simulink model "Air_Drag"  (R2023b)
settings: Solver=VariableStepAuto  StartTime=0.0  StopTime=T_1orbit  RelTol=1e-6
values from neighbouring files (symbols this model uses):
  a = 6939    [Air_Drag_script.m]    (also in main.m = 6939.063; main_group24.m = 6978)
  A0 = eye(3)    [Air_Drag_script.m]
  A1 = 6e-2    (= 0.06)    [Air_Drag_script.m]
  A10 = 12e-2    (= 0.12)    [Air_Drag_script.m]
  A2 = 6e-2    (= 0.06)    [Air_Drag_script.m]
  A3 = 4e-2    (= 0.04)    [Air_Drag_script.m]
  A4 = 6e-2    (= 0.06)    [Air_Drag_script.m]
  A5 = 6e-2    (= 0.06)    [Air_Drag_script.m]
  A6 = 4e-2    (= 0.04)    [Air_Drag_script.m]
  A7 = 12e-2    (= 0.12)    [Air_Drag_script.m]
  A8 = 12e-2    (= 0.12)    [Air_Drag_script.m]
  A9 = 12e-2    (= 0.12)    [Air_Drag_script.m]
  cd = 2.2    [Air_Drag_script.m]
  e = 0    [Air_Drag_script.m]    (also in main.m = 0.001304; main_group24.m)
  i = deg2rad(97.5307)    [Air_Drag_script.m]    (also in main.m; main_group24.m = deg2rad(98))
  Ix = J(1,1)    [Air_Drag_script.m]    (also in data_mass.m = 0.0755003333333; main.m = 0.057749855; main_group24.m = 0.0755003333333)
  Iy = J(2,2)    [Air_Drag_script.m]    (also in data_mass.m = 0.0755003333333; main.m = 0.04143542; main_group24.m = 0.0755003333333)
  Iz = J(3,3)    [Air_Drag_script.m]    (also in data_mass.m = 0.055; main.m = 0.024624309; main_group24.m = 0.055)
  n = 0.0011    [Air_Drag_script.m]    (also in main.m = sqrt(mu/a^3); main_group24.m = sqrt(mu/a^3))
  n1 = [1 0 0]'    [Air_Drag_script.m]
  n10 = -n9    [Air_Drag_script.m]
  n2 = [0 1 0]'    [Air_Drag_script.m]
  n3 = [0 0 1]'    [Air_Drag_script.m]
  n4 = -n1    [Air_Drag_script.m]
  n5 = -n2    [Air_Drag_script.m]
  n6 = -n3    [Air_Drag_script.m]
  n7 = [1 0 0]'    [Air_Drag_script.m]
  n8 = -n7    [Air_Drag_script.m]
  n9 = [1 0 0]'    [Air_Drag_script.m]
  q0 = [ 1 1 1 1 ]'    [Air_Drag_script.m]    (also in main_group24.m = [0 0 0 1]')
  r1 = [10 0 0]'*1e-2    [Air_Drag_script.m]
  r10 = r9    [Air_Drag_script.m]
  r2 = [0,10,0]'*1e-2    [Air_Drag_script.m]
  r3 = [0,0,10]'*1e-2    [Air_Drag_script.m]
  r4 = -r1    [Air_Drag_script.m]
  r5 = -r2    [Air_Drag_script.m]
  r6 = -r3    [Air_Drag_script.m]
  r7 = [0,0,45]'*1e-2    [Air_Drag_script.m]
  r8 = r7    [Air_Drag_script.m]
  r9 = [0,0,-45]'*1e-2    [Air_Drag_script.m]
  rho_air = 1.65e-13    [Air_Drag_script.m]    (also in main_group24.m = 6.967e-13)
  w0 = [0 0 0]'    [Air_Drag_script.m]    (also in main.m = [wx0; wy0; wz0]; main_group24.m = [wx0; wy0; wz0])
  w_earth = [0 0 7.2921e-5]'    [Air_Drag_script.m]
libraries: matrix_library x12, vrlib x10
settings Model: Creator=hp  LastModifiedBy=hp

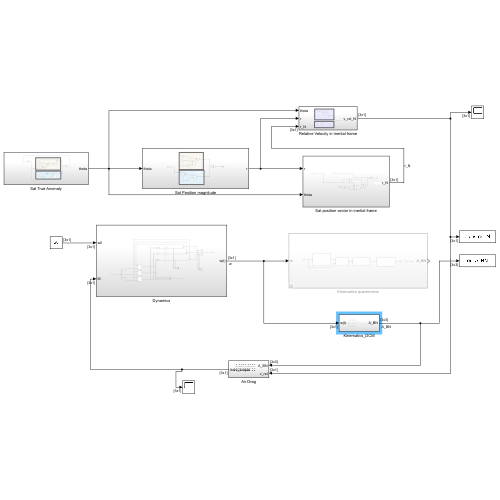
[thumbnail: Simulink's stored preview of the top-level diagram]
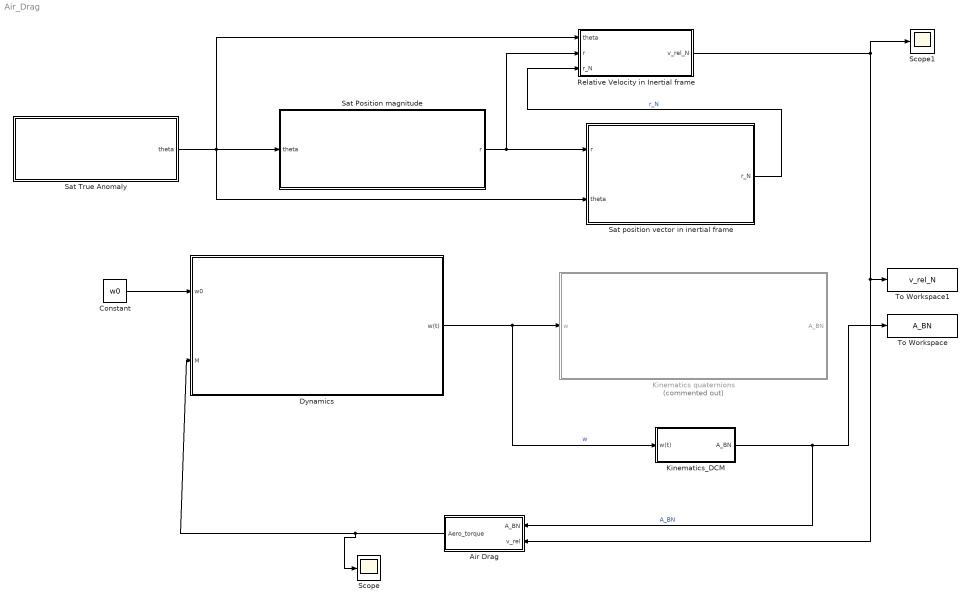
== system Air_Drag ==
  Air Drag : Subsystem
  Constant : Constant  Value=w0  VectorParams1D=off
  Dynamics : Subsystem
  Kinematics quaternions : Subsystem  Commented=on
  Kinematics_DCM : Subsystem
  Relative Velocity in Inertial frame : Subsystem
  Sat Position magnitude : Subsystem
  Sat True Anomaly : Subsystem
  Sat position vector in inertial frame : Subsystem
  Scope : Scope
  Scope1 : Scope
  To Workspace : ToWorkspace  VariableName=A_BN  SaveFormat=Timeseries  SampleTime=-1
  To Workspace1 : ToWorkspace  VariableName=v_rel_N  SaveFormat=Timeseries  SampleTime=-1
  wires:
  Sat True Anomaly/1(theta) -> Relative Velocity in Inertial frame/1(theta), Sat position vector in inertial frame/2(theta), Sat Position magnitude/1(theta)
  Sat Position magnitude/1(r) -> Sat position vector in inertial frame/1(r), Relative Velocity in Inertial frame/2(r)
  Sat position vector in inertial frame/1(r_N) -> Relative Velocity in Inertial frame/3(r_N)  "r_N"
  Dynamics/1(w(t)) -> Kinematics_DCM/1(w(t)), Kinematics quaternions/1(w)  "w"
  Constant/1 -> Dynamics/1(w0)
  Relative Velocity in Inertial frame/1(v_rel_N) -> To Workspace1/1, Air Drag/2(v_rel), Scope1/1
  Air Drag/1(Aero_torque) -> Scope/1, Dynamics/2(M)
  Kinematics_DCM/1(A_BN) -> Air Drag/1(A_BN), To Workspace/1  "A_BN"

== system Air_Drag/Air Drag ==
  A_BN : Inport
  v_rel : Inport  Port=2
  Sum of Elements : Sum  Inputs=++++++++++
  T1 : Subsystem
  T10 : Subsystem
  T2 : Subsystem
  T3 : Subsystem
  T4 : Subsystem
  T5 : Subsystem
  T6 : Subsystem
  T7 : Subsystem
  T8 : Subsystem
  T9 : Subsystem
  Aero_torque : Outport
  wires:
  Sum of Elements/1 -> Aero_torque/1
  v_rel/1 -> T10/1(v_rel_N), T7/1(v_rel_N), T6/1(v_rel_N), T2/1(v_rel_N), T1/1(v_rel_N), T3/1(v_rel_N), T4/1(v_rel_N), T5/1(v_rel_N), T8/1(v_rel_N), T9/1(v_rel_N)  "v_rel_N"
  A_BN/1 -> T8/2(A_BN), T5/2(A_BN), T4/2(A_BN), T2/2(A_BN), T1/2(A_BN), T3/2(A_BN), T6/2(A_BN), T7/2(A_BN), T9/2(A_BN), T10/2(A_BN)
  T1/1(Out1) -> Sum of Elements/1
  T2/1(Out1) -> Sum of Elements/2
  T3/1(Out1) -> Sum of Elements/3
  T4/1(Out1) -> Sum of Elements/4
  T5/1(Out1) -> Sum of Elements/5
  T6/1(Out1) -> Sum of Elements/6
  T7/1(Out1) -> Sum of Elements/7
  T8/1(Out1) -> Sum of Elements/8
  T9/1(Out1) -> Sum of Elements/9
  T10/1(Out1) -> Sum of Elements/10

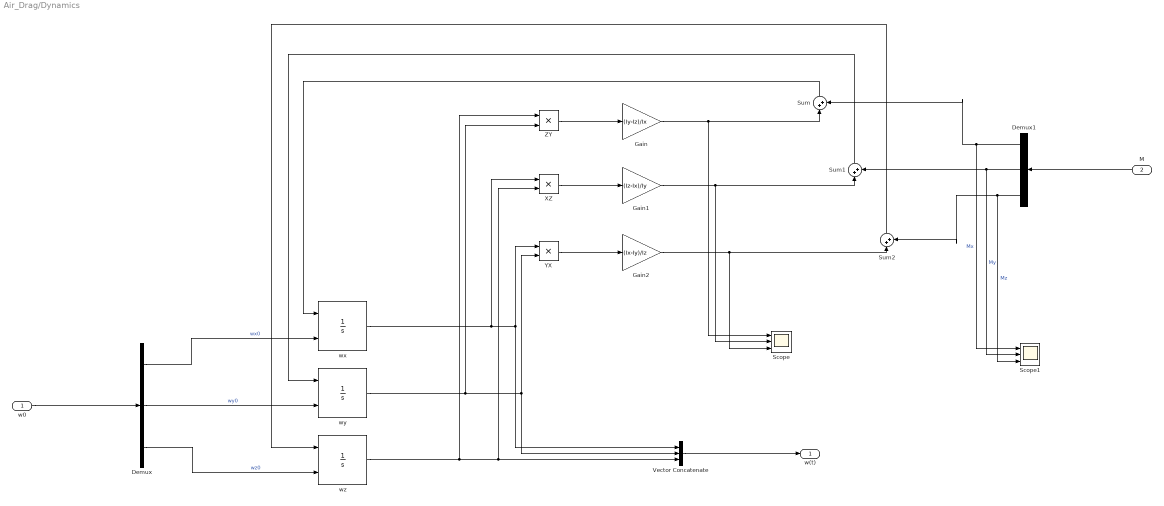
== system Air_Drag/Dynamics ==
  w0 : Inport
  M : Inport  Port=2
  Demux : Demux  Outputs=3
  Demux1 : Demux  Outputs=3
  Gain : Gain  Gain=(Iy-Iz)/Ix
  Gain1 : Gain  Gain=(Iz-Ix)/Iy
  Gain2 : Gain  Gain=(Ix-Iy)/Iz
  Scope : Scope  NumInputPorts=3
  Scope1 : Scope  NumInputPorts=3
  Sum : Sum  Inputs=|++
  Sum1 : Sum  Inputs=|++
  Sum2 : Sum  Inputs=|++
  Vector Concatenate : Concatenate  NumInputs=3  Mode=Multidimensional array
  XZ : Product
  YX : Product
  ZY : Product
  wx : Integrator  InitialConditionSource=external
  wy : Integrator  InitialConditionSource=external
  wz : Integrator  InitialConditionSource=external
  w(t) : Outport
  wires:
  XZ/1 -> Gain1/1
  Demux/2 -> wy/2  "wy0"
  wx/1 -> XZ/1, Vector Concatenate/1, YX/1
  w0/1 -> Demux/1
  wy/1 -> Vector Concatenate/2, YX/2, ZY/2
  Demux/1 -> wx/2  "wx0"
  wz/1 -> ZY/1, Vector Concatenate/3, XZ/2
  YX/1 -> Gain2/1
  Demux/3 -> wz/2  "wz0"
  ZY/1 -> Gain/1
  Vector Concatenate/1 -> w(t)/1
  Gain2/1 -> Scope/3, Sum2/1
  Gain1/1 -> Scope/2, Sum1/1
  Gain/1 -> Scope/1, Sum/1
  Sum/1 -> wx/1
  Sum1/1 -> wy/1
  Sum2/1 -> wz/1
  Demux1/1 -> Scope1/1, Sum/2  "Mx"
  Demux1/2 -> Scope1/2, Sum1/2  "My"
  Demux1/3 -> Sum2/2, Scope1/3  "Mz"
  M/1 -> Demux1/1

== system Air_Drag/Kinematics quaternions ==
  w : Inport
  A_BN from q_vect : MATLAB Function  TreatAsAtomicUnit=on
  Create Omega Matrix : Subsystem
  Kinematics_quaternions : Subsystem
  Normalizer : Subsystem
  w_at_matrix : Subsystem
  A_BN : Outport
  wires:
  Kinematics_quaternions/1(q_vect) -> A_BN from q_vect/1(q_vect)
  A_BN from q_vect/1(A_BN) -> Normalizer/1(A_BN)
  w/1 -> Create Omega Matrix/2(w), w_at_matrix/1(w(t))
  Create Omega Matrix/1(Omega) -> Kinematics_quaternions/1(Omega)  "Omega"
  w_at_matrix/1("[-w^]") -> Create Omega Matrix/1("[w^]")  "[-w^]"
  Normalizer/1(Out1) -> A_BN/1

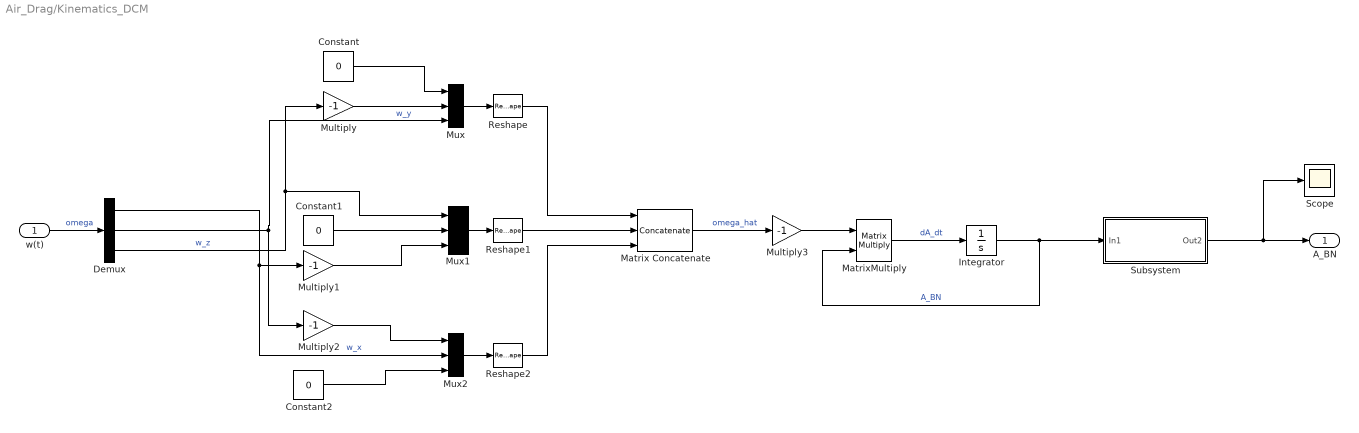
== system Air_Drag/Kinematics_DCM ==
  w(t) : Inport
  Constant : Constant  Value=0
  Constant1 : Constant  Value=0
  Constant2 : Constant  Value=0
  Demux : Demux  Outputs=3
  Integrator : Integrator  InitialCondition=A0
  Matrix Concatenate : Concatenate  NumInputs=3  Mode=Multidimensional array
  MatrixMultiply : Product  Multiplication=Matrix(*)
  Multiply{,1..3} (4 alike) : Gain  Gain=-1
  Mux : Mux  Inputs=3
  Mux1 : Mux  Inputs=3
  Mux2 : Mux  Inputs=3
  Reshape : Reshape  OutputDimensionality=Row vector (2-D)
  Reshape1 : Reshape  OutputDimensionality=Row vector (2-D)
  Reshape2 : Reshape  OutputDimensionality=Row vector (2-D)
  Scope : Scope
  Subsystem : Subsystem
  A_BN : Outport
  wires:
  w(t)/1 -> Demux/1  "omega"
  MatrixMultiply/1 -> Integrator/1  "dA_dt"
  Matrix Concatenate/1 -> Multiply3/1  "omega_hat"
  Constant/1 -> Mux/1
  Demux/3 -> Mux1/1, Multiply/1  "w_z"
  Multiply/1 -> Mux/2
  Demux/2 -> Mux/3, Multiply2/1  "w_y"
  Constant1/1 -> Mux1/2
  Demux/1 -> Mux2/2, Multiply1/1  "w_x"
  Multiply1/1 -> Mux1/3
  Constant2/1 -> Mux2/3
  Multiply2/1 -> Mux2/1
  Mux/1 -> Reshape/1
  Mux1/1 -> Reshape1/1
  Mux2/1 -> Reshape2/1
  Multiply3/1 -> MatrixMultiply/1
  Reshape/1 -> Matrix Concatenate/1
  Reshape1/1 -> Matrix Concatenate/2
  Reshape2/1 -> Matrix Concatenate/3
  Integrator/1 -> Subsystem/1(In1), MatrixMultiply/2  "A_BN"
  Subsystem/1(Out2) -> Scope/1, A_BN/1

== system Air_Drag/Relative Velocity in Inertial frame ==
  note: V_orbit
  note: V_atmosphere
  theta : Inport
  r : Inport  Port=2
  r_N : Inport  Port=3
  Constant : Constant  Value=n
  Constant3 : Constant  Value=w_earth  VectorParams1D=off
  Cos : Trigonometry  Operator=cos
  Cross Product : matrix_library/Cross Product
  Gain : Gain  Gain=-1
  Gain1 : Gain  Gain=cos(i)
  Gain2 : Gain  Gain=sin(i)
  Product : Product  Inputs=3
  Sin : Trigonometry
  Sum1 : Sum  Inputs=+-
  Vector Concatenate : Concatenate  NumInputs=3
  v_rel_N : Outport
  wires:
  Sum1/1 -> v_rel_N/1
  r_N/1 -> Cross Product/2
  Constant3/1 -> Cross Product/1
  Product/1 -> Sum1/1
  Cross Product/1 -> Sum1/2
  r/1 -> Product/2
  Constant/1 -> Product/3
  theta/1 -> Cos/1, Sin/1
  Gain/1 -> Vector Concatenate/1
  Gain1/1 -> Vector Concatenate/2
  Gain2/1 -> Vector Concatenate/3
  Cos/1 -> Gain2/1, Gain1/1
  Sin/1 -> Gain/1
  Vector Concatenate/1 -> Product/1

== system Air_Drag/Sat Position magnitude ==
  note: 1+e cos(theta)
  note: a(1-e^2)
  note: Denominator
  note: Numerator
  theta : Inport
  Constant : Constant  Value=a
  Constant1 : Constant
  Constant3 : Constant  Value=e
  Constant4 : Constant
  Constant5 : Constant  Value=e
  Cos : Trigonometry  Operator=cos
  Divide : Product  Inputs=*/
  Product : Product
  Product1 : Product
  Square1 : Math  Operator=square
  Sum : Sum
  Sum1 : Sum  Inputs=+-
  r : Outport
  wires:
  Product1/1 -> Sum/1
  Sum1/1 -> Product/2
  Constant1/1 -> Sum1/1
  Sum/1 -> Divide/2
  Square1/1 -> Sum1/2
  Constant3/1 -> Product1/2
  Constant4/1 -> Sum/2
  Constant/1 -> Product/1
  Constant5/1 -> Square1/1
  Cos/1 -> Product1/1
  Product/1 -> Divide/1
  theta/1 -> Cos/1
  Divide/1 -> r/1

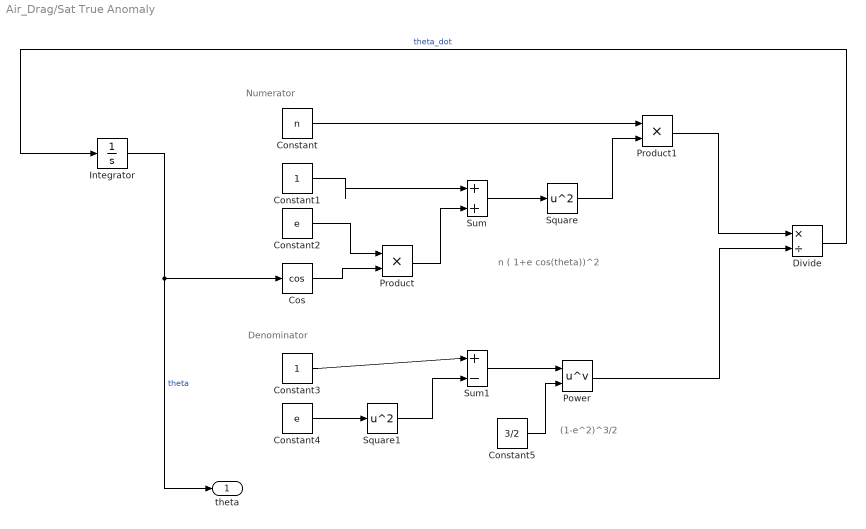
== system Air_Drag/Sat True Anomaly ==
  note: (1-e^2)^3/2
  note: n ( 1+e cos(theta))^2
  note: Denominator
  note: Numerator
  Constant : Constant  Value=n
  Constant1 : Constant
  Constant2 : Constant  Value=e
  Constant3 : Constant
  Constant4 : Constant  Value=e
  Constant5 : Constant  Value=3/2
  Cos : Trigonometry  Operator=cos
  Divide : Product  Inputs=*/
  Integrator : Integrator
  Power : Math  Operator=pow
  Product : Product
  Product1 : Product
  Square : Math  Operator=square
  Square1 : Math  Operator=square
  Sum : Sum  Inputs=|++
  Sum1 : Sum  Inputs=|+-
  theta : Outport
  wires:
  Sum/1 -> Square/1
  Integrator/1 -> theta/1, Cos/1  "theta"
  Square/1 -> Product1/2
  Constant5/1 -> Power/2
  Constant3/1 -> Sum1/1
  Product1/1 -> Divide/1
  Constant/1 -> Product1/1
  Divide/1 -> Integrator/1  "theta_dot"
  Square1/1 -> Sum1/2
  Product/1 -> Sum/2
  Power/1 -> Divide/2
  Constant1/1 -> Sum/1
  Constant2/1 -> Product/1
  Constant4/1 -> Square1/1
  Cos/1 -> Product/2
  Sum1/1 -> Power/1

== system Air_Drag/Sat position vector in inertial frame ==
  note: r_N = r [cos(theta)
      | 		sin(theta)cos(i)
      | 		sin(theta)sin(i)]
  r : Inport
  theta : Inport  Port=2
  Cos : Trigonometry  Operator=cos
  Cos1 : Trigonometry  Operator=cos
  Orbit Inclination : Constant  Value=i
  Product : Product
  Product1 : Product
  Product2 : Product
  Sin : Trigonometry
  Sin1 : Trigonometry
  Vector Concatenate : Concatenate  NumInputs=3  Mode=Multidimensional array
  r_N : Outport
  wires:
  Sin/1 -> Product1/1, Product/1
  Product/1 -> Vector Concatenate/2
  Sin1/1 -> Product1/2
  r/1 -> Product2/1
  Orbit Inclination/1 -> Sin1/1, Cos1/1
  Vector Concatenate/1 -> Product2/2
  theta/1 -> Cos/1, Sin/1
  Cos/1 -> Vector Concatenate/1
  Cos1/1 -> Product/2
  Product1/1 -> Vector Concatenate/3
  Product2/1 -> r_N/1

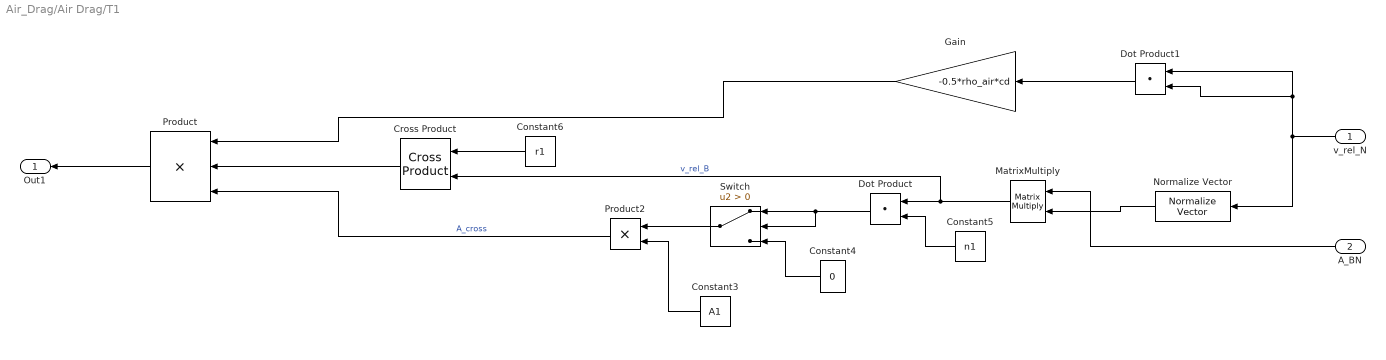
== system Air_Drag/Air Drag/T1 ==
  v_rel_N : Inport
  A_BN : Inport  Port=2
  Constant3 : Constant  Value=A1
  Constant4 : Constant  Value=0
  Constant5 : Constant  Value=n1  VectorParams1D=off
  Constant6 : Constant  Value=r1  VectorParams1D=off
  Cross Product : matrix_library/Cross Product
  Dot Product : DotProduct  OutDataTypeStr=Inherit: Inherit via internal rule
  Dot Product1 : DotProduct  OutDataTypeStr=Inherit: Inherit via internal rule
  Gain : Gain  Gain=-0.5*rho_air*cd
  MatrixMultiply : Product  Multiplication=Matrix(*)
  Normalize Vector : vrlib/Utilities/Normalize Vector  maxzero=0
  Product : Product  Inputs=3
  Product2 : Product
  Switch : Switch  Criteria=u2 > Threshold  SaturateOnIntegerOverflow=off  InputSameDT=off
  Out1 : Outport
  wires:
  MatrixMultiply/1 -> Cross Product/2, Dot Product/1  "v_rel_B"
  Constant4/1 -> Switch/3
  Dot Product/1 -> Switch/1, Switch/2
  v_rel_N/1 -> Dot Product1/2, Dot Product1/1, Normalize Vector/1
  Switch/1 -> Product2/1
  Constant6/1 -> Cross Product/1
  Constant5/1 -> Dot Product/2
  Constant3/1 -> Product2/2
  Gain/1 -> Product/1
  Dot Product1/1 -> Gain/1
  Cross Product/1 -> Product/2
  Product2/1 -> Product/3  "A_cross"
  Normalize Vector/1 -> MatrixMultiply/2
  A_BN/1 -> MatrixMultiply/1
  Product/1 -> Out1/1

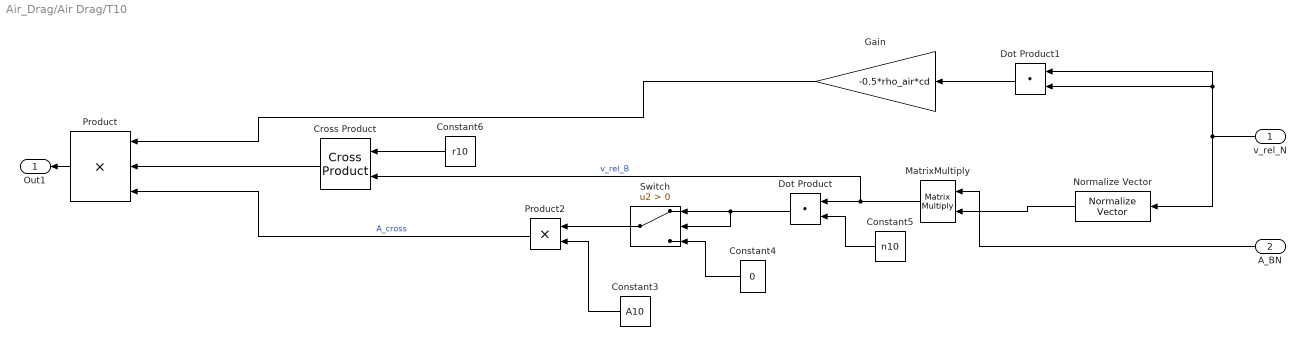
== system Air_Drag/Air Drag/T10 ==
  v_rel_N : Inport
  A_BN : Inport  Port=2
  Constant3 : Constant  Value=A10
  Constant4 : Constant  Value=0
  Constant5 : Constant  Value=n10  VectorParams1D=off
  Constant6 : Constant  Value=r10  VectorParams1D=off
  Cross Product : matrix_library/Cross Product
  Dot Product : DotProduct  OutDataTypeStr=Inherit: Inherit via internal rule
  Dot Product1 : DotProduct  OutDataTypeStr=Inherit: Inherit via internal rule
  Gain : Gain  Gain=-0.5*rho_air*cd
  MatrixMultiply : Product  Multiplication=Matrix(*)
  Normalize Vector : vrlib/Utilities/Normalize Vector  maxzero=0
  Product : Product  Inputs=3
  Product2 : Product
  Switch : Switch  Criteria=u2 > Threshold  SaturateOnIntegerOverflow=off  InputSameDT=off
  Out1 : Outport
  wires:
  Product/1 -> Out1/1
  A_BN/1 -> MatrixMultiply/1
  Normalize Vector/1 -> MatrixMultiply/2
  Product2/1 -> Product/3  "A_cross"
  Cross Product/1 -> Product/2
  Dot Product1/1 -> Gain/1
  Gain/1 -> Product/1
  Constant3/1 -> Product2/2
  Constant5/1 -> Dot Product/2
  Constant6/1 -> Cross Product/1
  Switch/1 -> Product2/1
  v_rel_N/1 -> Dot Product1/2, Dot Product1/1, Normalize Vector/1
  Dot Product/1 -> Switch/2, Switch/1
  Constant4/1 -> Switch/3
  MatrixMultiply/1 -> Dot Product/1, Cross Product/2  "v_rel_B"

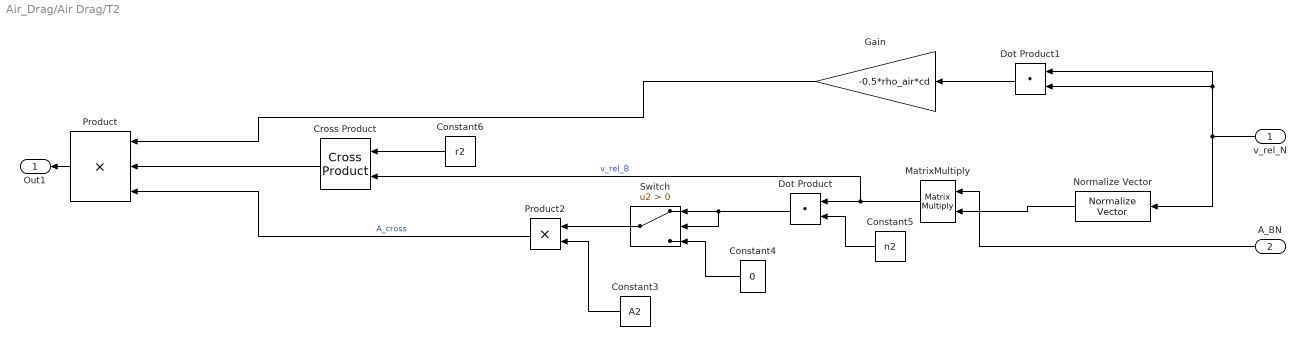
== system Air_Drag/Air Drag/T2 ==
  v_rel_N : Inport
  A_BN : Inport  Port=2
  Constant3 : Constant  Value=A2
  Constant4 : Constant  Value=0
  Constant5 : Constant  Value=n2  VectorParams1D=off
  Constant6 : Constant  Value=r2  VectorParams1D=off
  Cross Product : matrix_library/Cross Product
  Dot Product : DotProduct  OutDataTypeStr=Inherit: Inherit via internal rule
  Dot Product1 : DotProduct  OutDataTypeStr=Inherit: Inherit via internal rule
  Gain : Gain  Gain=-0.5*rho_air*cd
  MatrixMultiply : Product  Multiplication=Matrix(*)
  Normalize Vector : vrlib/Utilities/Normalize Vector  maxzero=0
  Product : Product  Inputs=3
  Product2 : Product
  Switch : Switch  Criteria=u2 > Threshold  SaturateOnIntegerOverflow=off  InputSameDT=off
  Out1 : Outport
  wires:
  Product/1 -> Out1/1
  A_BN/1 -> MatrixMultiply/1
  Normalize Vector/1 -> MatrixMultiply/2
  Product2/1 -> Product/3  "A_cross"
  Cross Product/1 -> Product/2
  Dot Product1/1 -> Gain/1
  Gain/1 -> Product/1
  Constant3/1 -> Product2/2
  Constant5/1 -> Dot Product/2
  Constant6/1 -> Cross Product/1
  Switch/1 -> Product2/1
  v_rel_N/1 -> Dot Product1/2, Dot Product1/1, Normalize Vector/1
  Dot Product/1 -> Switch/2, Switch/1
  Constant4/1 -> Switch/3
  MatrixMultiply/1 -> Dot Product/1, Cross Product/2  "v_rel_B"

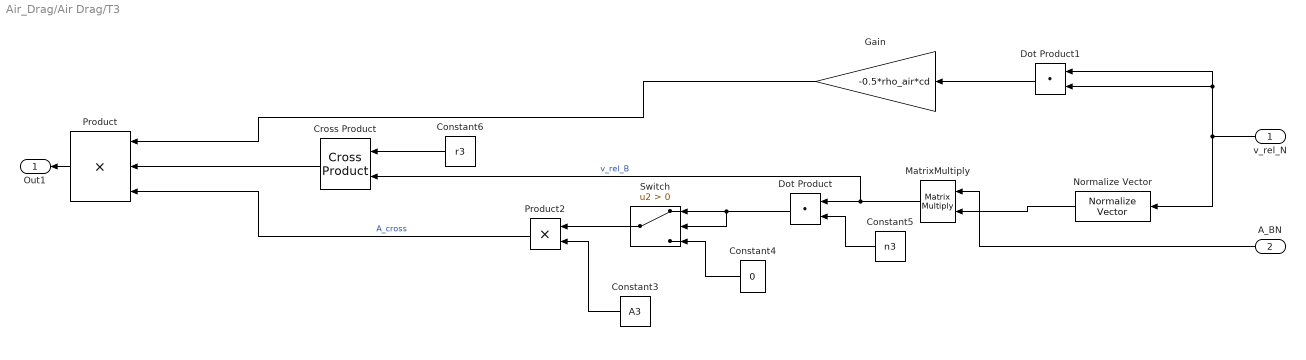
== system Air_Drag/Air Drag/T3 ==
  v_rel_N : Inport
  A_BN : Inport  Port=2
  Constant3 : Constant  Value=A3
  Constant4 : Constant  Value=0
  Constant5 : Constant  Value=n3  VectorParams1D=off
  Constant6 : Constant  Value=r3  VectorParams1D=off
  Cross Product : matrix_library/Cross Product
  Dot Product : DotProduct  OutDataTypeStr=Inherit: Inherit via internal rule
  Dot Product1 : DotProduct  OutDataTypeStr=Inherit: Inherit via internal rule
  Gain : Gain  Gain=-0.5*rho_air*cd
  MatrixMultiply : Product  Multiplication=Matrix(*)
  Normalize Vector : vrlib/Utilities/Normalize Vector  maxzero=0
  Product : Product  Inputs=3
  Product2 : Product
  Switch : Switch  Criteria=u2 > Threshold  SaturateOnIntegerOverflow=off  InputSameDT=off
  Out1 : Outport
  wires:
  MatrixMultiply/1 -> Cross Product/2, Dot Product/1  "v_rel_B"
  Constant4/1 -> Switch/3
  Dot Product/1 -> Switch/2, Switch/1
  v_rel_N/1 -> Dot Product1/2, Dot Product1/1, Normalize Vector/1
  Switch/1 -> Product2/1
  Constant6/1 -> Cross Product/1
  Constant5/1 -> Dot Product/2
  Constant3/1 -> Product2/2
  Gain/1 -> Product/1
  Dot Product1/1 -> Gain/1
  Cross Product/1 -> Product/2
  Product2/1 -> Product/3  "A_cross"
  Normalize Vector/1 -> MatrixMultiply/2
  A_BN/1 -> MatrixMultiply/1
  Product/1 -> Out1/1

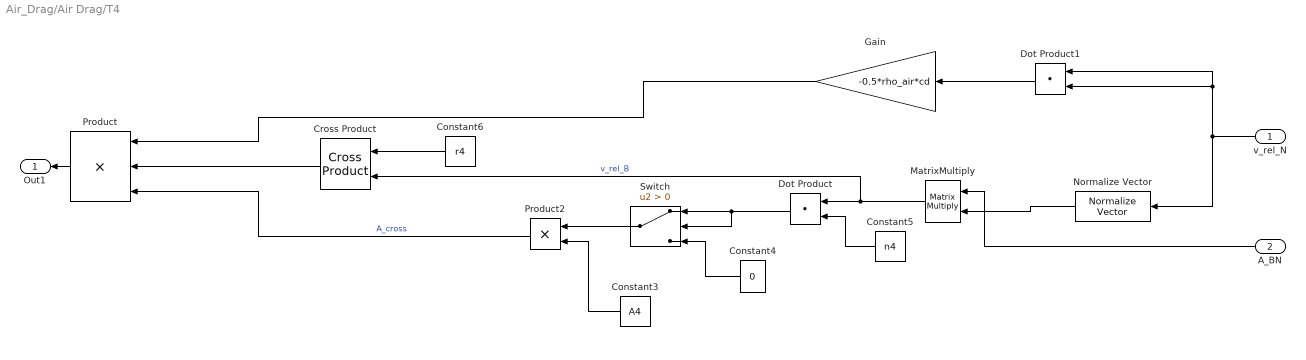
== system Air_Drag/Air Drag/T4 ==
  v_rel_N : Inport
  A_BN : Inport  Port=2
  Constant3 : Constant  Value=A4
  Constant4 : Constant  Value=0
  Constant5 : Constant  Value=n4  VectorParams1D=off
  Constant6 : Constant  Value=r4  VectorParams1D=off
  Cross Product : matrix_library/Cross Product
  Dot Product : DotProduct  OutDataTypeStr=Inherit: Inherit via internal rule
  Dot Product1 : DotProduct  OutDataTypeStr=Inherit: Inherit via internal rule
  Gain : Gain  Gain=-0.5*rho_air*cd
  MatrixMultiply : Product  Multiplication=Matrix(*)
  Normalize Vector : vrlib/Utilities/Normalize Vector  maxzero=0
  Product : Product  Inputs=3
  Product2 : Product
  Switch : Switch  Criteria=u2 > Threshold  SaturateOnIntegerOverflow=off  InputSameDT=off
  Out1 : Outport
  wires:
  Product/1 -> Out1/1
  A_BN/1 -> MatrixMultiply/1
  Normalize Vector/1 -> MatrixMultiply/2
  Product2/1 -> Product/3  "A_cross"
  Cross Product/1 -> Product/2
  Dot Product1/1 -> Gain/1
  Gain/1 -> Product/1
  Constant3/1 -> Product2/2
  Constant5/1 -> Dot Product/2
  Constant6/1 -> Cross Product/1
  Switch/1 -> Product2/1
  Dot Product/1 -> Switch/2, Switch/1
  Constant4/1 -> Switch/3
  MatrixMultiply/1 -> Dot Product/1, Cross Product/2  "v_rel_B"
  v_rel_N/1 -> Dot Product1/2, Dot Product1/1, Normalize Vector/1

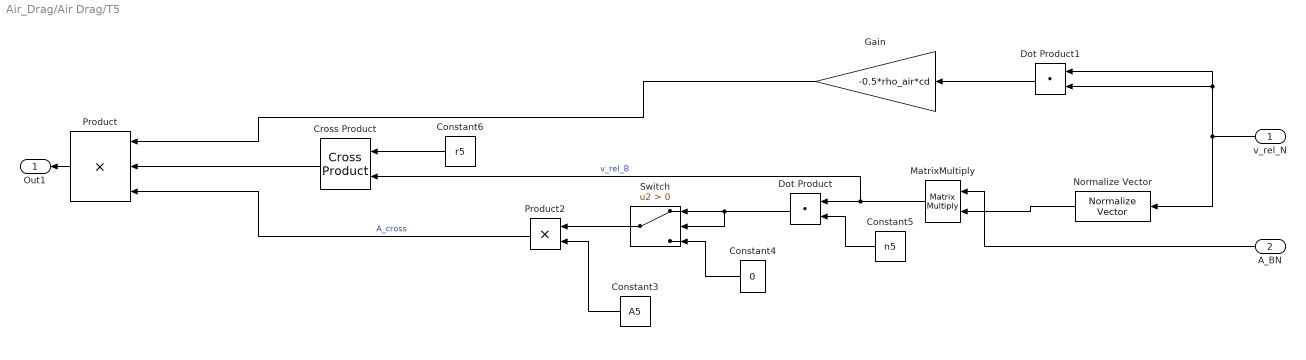
== system Air_Drag/Air Drag/T5 ==
  v_rel_N : Inport
  A_BN : Inport  Port=2
  Constant3 : Constant  Value=A5
  Constant4 : Constant  Value=0
  Constant5 : Constant  Value=n5  VectorParams1D=off
  Constant6 : Constant  Value=r5  VectorParams1D=off
  Cross Product : matrix_library/Cross Product
  Dot Product : DotProduct  OutDataTypeStr=Inherit: Inherit via internal rule
  Dot Product1 : DotProduct  OutDataTypeStr=Inherit: Inherit via internal rule
  Gain : Gain  Gain=-0.5*rho_air*cd
  MatrixMultiply : Product  Multiplication=Matrix(*)
  Normalize Vector : vrlib/Utilities/Normalize Vector  maxzero=0
  Product : Product  Inputs=3
  Product2 : Product
  Switch : Switch  Criteria=u2 > Threshold  SaturateOnIntegerOverflow=off  InputSameDT=off
  Out1 : Outport
  wires:
  MatrixMultiply/1 -> Cross Product/2, Dot Product/1  "v_rel_B"
  Constant4/1 -> Switch/3
  Dot Product/1 -> Switch/2, Switch/1
  Switch/1 -> Product2/1
  Constant6/1 -> Cross Product/1
  Constant5/1 -> Dot Product/2
  Constant3/1 -> Product2/2
  Gain/1 -> Product/1
  Dot Product1/1 -> Gain/1
  Cross Product/1 -> Product/2
  Product2/1 -> Product/3  "A_cross"
  Normalize Vector/1 -> MatrixMultiply/2
  A_BN/1 -> MatrixMultiply/1
  Product/1 -> Out1/1
  v_rel_N/1 -> Dot Product1/2, Dot Product1/1, Normalize Vector/1

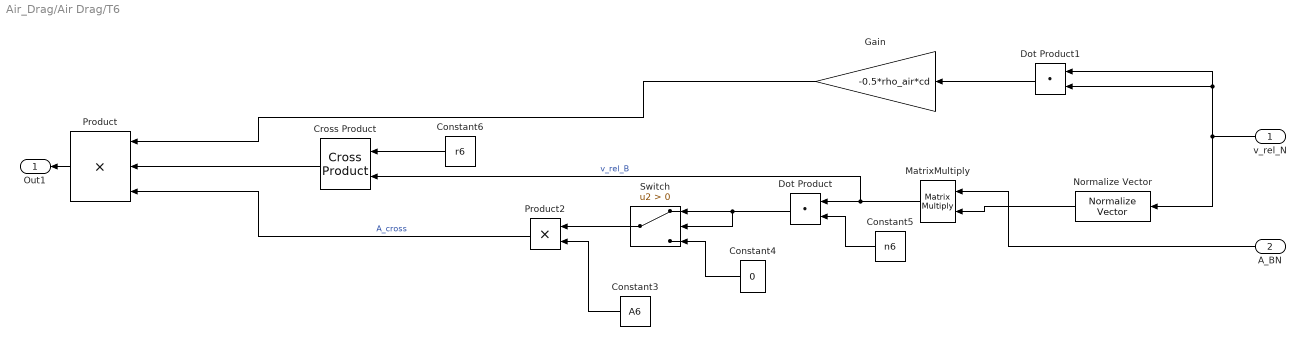
== system Air_Drag/Air Drag/T6 ==
  v_rel_N : Inport
  A_BN : Inport  Port=2
  Constant3 : Constant  Value=A6
  Constant4 : Constant  Value=0
  Constant5 : Constant  Value=n6  VectorParams1D=off
  Constant6 : Constant  Value=r6  VectorParams1D=off
  Cross Product : matrix_library/Cross Product
  Dot Product : DotProduct  OutDataTypeStr=Inherit: Inherit via internal rule
  Dot Product1 : DotProduct  OutDataTypeStr=Inherit: Inherit via internal rule
  Gain : Gain  Gain=-0.5*rho_air*cd
  MatrixMultiply : Product  Multiplication=Matrix(*)
  Normalize Vector : vrlib/Utilities/Normalize Vector  maxzero=0
  Product : Product  Inputs=3
  Product2 : Product
  Switch : Switch  Criteria=u2 > Threshold  SaturateOnIntegerOverflow=off  InputSameDT=off
  Out1 : Outport
  wires:
  Product/1 -> Out1/1
  A_BN/1 -> MatrixMultiply/1
  Normalize Vector/1 -> MatrixMultiply/2
  Product2/1 -> Product/3  "A_cross"
  Cross Product/1 -> Product/2
  Dot Product1/1 -> Gain/1
  Gain/1 -> Product/1
  Constant3/1 -> Product2/2
  Constant5/1 -> Dot Product/2
  Constant6/1 -> Cross Product/1
  Switch/1 -> Product2/1
  v_rel_N/1 -> Dot Product1/2, Dot Product1/1, Normalize Vector/1
  Dot Product/1 -> Switch/2, Switch/1
  Constant4/1 -> Switch/3
  MatrixMultiply/1 -> Dot Product/1, Cross Product/2  "v_rel_B"

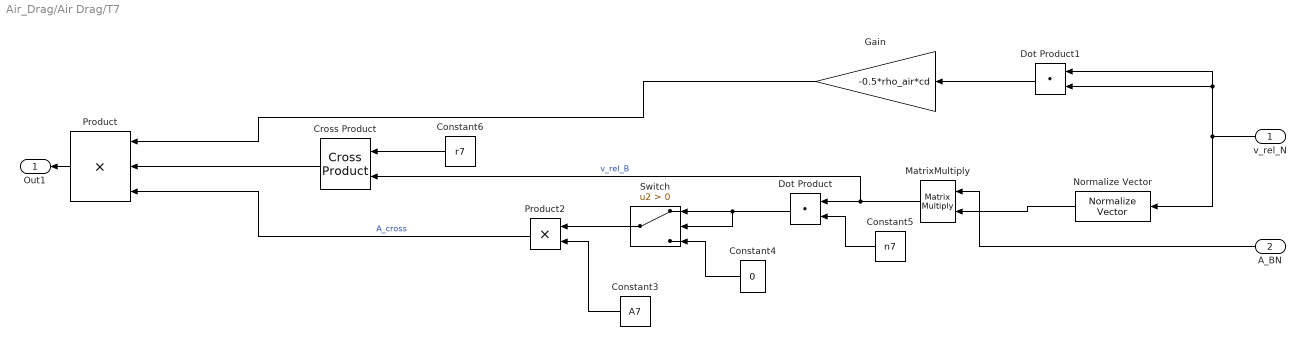
== system Air_Drag/Air Drag/T7 ==
  v_rel_N : Inport
  A_BN : Inport  Port=2
  Constant3 : Constant  Value=A7
  Constant4 : Constant  Value=0
  Constant5 : Constant  Value=n7  VectorParams1D=off
  Constant6 : Constant  Value=r7  VectorParams1D=off
  Cross Product : matrix_library/Cross Product
  Dot Product : DotProduct  OutDataTypeStr=Inherit: Inherit via internal rule
  Dot Product1 : DotProduct  OutDataTypeStr=Inherit: Inherit via internal rule
  Gain : Gain  Gain=-0.5*rho_air*cd
  MatrixMultiply : Product  Multiplication=Matrix(*)
  Normalize Vector : vrlib/Utilities/Normalize Vector  maxzero=0
  Product : Product  Inputs=3
  Product2 : Product
  Switch : Switch  Criteria=u2 > Threshold  SaturateOnIntegerOverflow=off  InputSameDT=off
  Out1 : Outport
  wires:
  MatrixMultiply/1 -> Cross Product/2, Dot Product/1  "v_rel_B"
  Constant4/1 -> Switch/3
  Dot Product/1 -> Switch/2, Switch/1
  v_rel_N/1 -> Dot Product1/2, Dot Product1/1, Normalize Vector/1
  Switch/1 -> Product2/1
  Constant6/1 -> Cross Product/1
  Constant5/1 -> Dot Product/2
  Constant3/1 -> Product2/2
  Gain/1 -> Product/1
  Dot Product1/1 -> Gain/1
  Cross Product/1 -> Product/2
  Product2/1 -> Product/3  "A_cross"
  Normalize Vector/1 -> MatrixMultiply/2
  A_BN/1 -> MatrixMultiply/1
  Product/1 -> Out1/1

== system Air_Drag/Air Drag/T8 ==
  v_rel_N : Inport
  A_BN : Inport  Port=2
  Constant3 : Constant  Value=A8
  Constant4 : Constant  Value=0
  Constant5 : Constant  Value=n8  VectorParams1D=off
  Constant6 : Constant  Value=r8  VectorParams1D=off
  Cross Product : matrix_library/Cross Product
  Dot Product : DotProduct  OutDataTypeStr=Inherit: Inherit via internal rule
  Dot Product1 : DotProduct  OutDataTypeStr=Inherit: Inherit via internal rule
  Gain : Gain  Gain=-0.5*rho_air*cd
  MatrixMultiply : Product  Multiplication=Matrix(*)
  Normalize Vector : vrlib/Utilities/Normalize Vector  maxzero=0
  Product : Product  Inputs=3
  Product2 : Product
  Switch : Switch  Criteria=u2 > Threshold  SaturateOnIntegerOverflow=off  InputSameDT=off
  Out1 : Outport
  wires:
  Product/1 -> Out1/1
  A_BN/1 -> MatrixMultiply/1
  Normalize Vector/1 -> MatrixMultiply/2
  Product2/1 -> Product/3  "A_cross"
  Cross Product/1 -> Product/2
  Dot Product1/1 -> Gain/1
  Gain/1 -> Product/1
  Constant3/1 -> Product2/2
  Constant5/1 -> Dot Product/2
  Constant6/1 -> Cross Product/1
  Switch/1 -> Product2/1
  v_rel_N/1 -> Dot Product1/2, Dot Product1/1, Normalize Vector/1
  Dot Product/1 -> Switch/2, Switch/1
  Constant4/1 -> Switch/3
  MatrixMultiply/1 -> Dot Product/1, Cross Product/2  "v_rel_B"

== system Air_Drag/Air Drag/T9 ==
  v_rel_N : Inport
  A_BN : Inport  Port=2
  Constant3 : Constant  Value=A9
  Constant4 : Constant  Value=0
  Constant5 : Constant  Value=n9  VectorParams1D=off
  Constant6 : Constant  Value=r9  VectorParams1D=off
  Cross Product : matrix_library/Cross Product
  Dot Product : DotProduct  OutDataTypeStr=Inherit: Inherit via internal rule
  Dot Product1 : DotProduct  OutDataTypeStr=Inherit: Inherit via internal rule
  Gain : Gain  Gain=-0.5*rho_air*cd
  MatrixMultiply : Product  Multiplication=Matrix(*)
  Normalize Vector : vrlib/Utilities/Normalize Vector  maxzero=0
  Product : Product  Inputs=3
  Product2 : Product
  Switch : Switch  Criteria=u2 > Threshold  SaturateOnIntegerOverflow=off  InputSameDT=off
  Out1 : Outport
  wires:
  MatrixMultiply/1 -> Cross Product/2, Dot Product/1  "v_rel_B"
  Constant4/1 -> Switch/3
  Dot Product/1 -> Switch/2, Switch/1
  v_rel_N/1 -> Dot Product1/2, Dot Product1/1, Normalize Vector/1
  Switch/1 -> Product2/1
  Constant6/1 -> Cross Product/1
  Constant5/1 -> Dot Product/2
  Constant3/1 -> Product2/2
  Gain/1 -> Product/1
  Dot Product1/1 -> Gain/1
  Cross Product/1 -> Product/2
  Product2/1 -> Product/3  "A_cross"
  Normalize Vector/1 -> MatrixMultiply/2
  A_BN/1 -> MatrixMultiply/1
  Product/1 -> Out1/1

== system Air_Drag/Kinematics quaternions/Create Omega Matrix ==
  "[w^]" : Inport
  w : Inport  Port=2
  " Col added" : Concatenate  Mode=Multidimensional array  ConcatenateDimension=2
  " Row added" : Concatenate  Mode=Multidimensional array
  Constant : Constant  Value=0
  Gain : Gain  Gain=-1
  Transpose : Math  Operator=transpose
  Vector Concatenate : Concatenate
  Omega : Outport
  wires:
  w/1 -> Transpose/1, Vector Concatenate/1
  Constant/1 -> Vector Concatenate/2
  Transpose/1 -> Gain/1
  "[w^]"/1 -> " Row added"/1
  " Row added"/1 -> " Col added"/1
  Vector Concatenate/1 -> " Col added"/2
  Gain/1 -> " Row added"/2
  " Col added"/1 -> Omega/1

== system Air_Drag/Kinematics quaternions/Kinematics_quaternions ==
  Omega : Inport
  Constant : Constant  Value=q0  VectorParams1D=off
  Gain : Gain  Gain=0.5
  Integrator : Integrator  InitialConditionSource=external  InitialCondition=q0
  Omega*q(t) : Product  Multiplication=Matrix(*)
  Scope : Scope
  q_vect : Outport
  wires:
  Gain/1 -> Scope/1, q_vect/1, Integrator/1
  Integrator/1 -> Omega*q(t)/2  "q(t)"
  Omega*q(t)/1 -> Gain/1
  Omega/1 -> Omega*q(t)/1
  Constant/1 -> Integrator/2

== system Air_Drag/Kinematics quaternions/Normalizer ==
  A_BN : Inport
  Gain : Gain  Gain=1.5
  Gain1 : Gain  Gain=0.5
  MatrixMultiply : Product  Multiplication=Matrix(*)
  MatrixMultiply1 : Product  Multiplication=Matrix(*)
  Sum : Sum  Inputs=+-
  Transpose : matrix_library/Transpose
  Out1 : Outport
  wires:
  A_BN/1 -> Transpose/1, MatrixMultiply/1, Gain/1, MatrixMultiply1/2
  Gain/1 -> Sum/1
  Sum/1 -> Out1/1
  Transpose/1 -> MatrixMultiply/2
  MatrixMultiply/1 -> MatrixMultiply1/1
  MatrixMultiply1/1 -> Gain1/1
  Gain1/1 -> Sum/2

== system Air_Drag/Kinematics quaternions/w_at_matrix ==
  w(t) : Inport
  Constant : Constant  Value=0  VectorParams1D=off
  Constant1 : Constant  Value=0
  Constant2 : Constant  Value=0
  Demux : Demux  Outputs=3
  Gain3 : Gain  Gain=-1
  Gain4 : Gain  Gain=-1
  Gain5 : Gain  Gain=-1
  Matrix Concatenate1 : Concatenate  NumInputs=3  Mode=Multidimensional array  ConcatenateDimension=2
  Mux1 : Mux  Inputs=3
  Mux2 : Mux  Inputs=3
  Mux3 : Mux  Inputs=3
  "[-w^]" : Outport
  wires:
  Demux/2 -> Mux1/3, Gain5/1  "wy"
  Gain3/1 -> Mux1/2
  Matrix Concatenate1/1 -> "[-w^]"/1
  Constant2/1 -> Mux3/3
  Demux/3 -> Mux2/1, Gain3/1  "wz"
  Constant1/1 -> Mux2/2
  Demux/1 -> Gain4/1, Mux3/2  "wx"
  Gain4/1 -> Mux2/3
  Mux1/1 -> Matrix Concatenate1/1
  Mux2/1 -> Matrix Concatenate1/2
  Gain5/1 -> Mux3/1
  Constant/1 -> Mux1/1
  Mux3/1 -> Matrix Concatenate1/3
  w(t)/1 -> Demux/1

== system Air_Drag/Kinematics_DCM/Subsystem ==
  In1 : Inport
  Matrix Multiply : Product  Multiplication=Matrix(*)
  Matrix Multiply1 : Product  Multiplication=Matrix(*)
  Multiply : Gain  Gain=3/2
  Multiply1 : Gain  Gain=1/2
  Subtract : Sum  Inputs=+-
  Transpose : Math  Operator=transpose
  Out2 : Outport
  wires:
  Subtract/1 -> Out2/1
  Multiply1/1 -> Subtract/2
  Matrix Multiply1/1 -> Multiply1/1
  Multiply/1 -> Subtract/1
  Transpose/1 -> Matrix Multiply/2
  Matrix Multiply/1 -> Matrix Multiply1/1
  In1/1 -> Matrix Multiply1/2, Matrix Multiply/1, Multiply/1, Transpose/1  "A"

== matlab function Air_Drag/Kinematics quaternions/A_BN from q_vect ==
  data: q_vect input; A_BN output
function A_BN = A_BN_form_q_vect(q_vect)
% function that provides the DCM A_BN from quaternions


q1 = q_vect(1);
q2 = q_vect(2);
q3 = q_vect(3);
q4 = q_vect(4);


    A_BN =[q1^2-q2^2-q3^2+q4^2 ,   2*(q1*q2+q3*q4)    ,   2*(q1*q3-q2*q4)
            2*(q1*q2-q3*q4)    , -q1^2+q2^2-q3^2+q4^2 ,   2*(q2*q3+q1*q4)
            2*(q1*q3+q2*q4)    ,   2*(q2*q3-q1*q4)    , -q1^2-q2^2+q3^2+q4^2];
